simulink model "ZynqBF_2tx_fpga_interface"  (R2018b)
settings: Solver=FixedStepDiscrete  StartTime=0.0  StopTime=inf  RelTol=1e-3  EnableMultiTasking=on
undefined symbols (not defined in the file): Fs, ip
libraries: gm_ZynqBF_2tx_fpga_lib x2, zynqlib x1
settings Model: SimulationMode=external  Creator=jason  LastModifiedBy=meyer
settings SolverCC: ConcurrentTasks=on  PositivePriorityOrder=on
settings DataIOCC: SaveOutput=off  SaveTime=off
settings OptimizationCC: BlockReduction=off  ConditionallyExecuteInputs=off  EnhancedBackFolding=on  PassReuseOutputArgsAs=Individual arguments  MaxStackSize=64  OptimizeBlockOrder=speed  DifferentSizesBufferReuse=on  OptimizationCustomize=off
settings DebuggingCC: AlgebraicLoopMsg=error  SingleTaskRateTransMsg=error  ParameterPrecisionLossMsg=none  ParameterTunabilityLossMsg=error  StrictBusMsg=ErrorOnBusTreatedAsVector
settings HardwareCC: ProdBitPerPointer=32  ProdBitPerSizeT=32  ProdBitPerPtrDiffT=32  ProdLargestAtomicInteger=Long  ProdLargestAtomicFloat=Double  ProdWordSize=32  ProdLongLongMode=on  ProdHWDeviceType=ARM Compatible->ARM Cortex  TargetLargestAtomicInteger=Long  TargetLargestAtomicFloat=Double  TargetIntDivRoundTo=Zero  TargetEndianess=LittleEndian  TargetHWDeviceType=ARM Compatible->ARM Cortex
settings SFSimCC: SimUseLocalCustomCode=off  MATLABDynamicMemAlloc=off
settings RTWCC: SystemTargetFile=ert.tlc  HardwareBoard=Xilinx Zynq-7000 Based IIO Radio  TLCOptions="-aInlineSetEventsForThisBaseRateFcn=TLC_FALSE -aSuppressMultiTaskScheduler=TLC_FALSE  -aRateBasedStepFcn=0"  TemplateMakefile=ert_default_tmf  GenerateReport=on  RTWUseLocalCustomCode=off  Toolchain=Linaro AArch32 Linux v6.3.1  IncludeHyperlinkInReport=on  LaunchReport=on  GenerateTraceInfo=on  GenerateTraceReport=on  GenerateTraceReportSl=on  GenerateTraceReportSf=on  GenerateTraceReportEml=on
settings CodeAppCC: ForceParamTrailComments=on  IgnoreCustomStorageClasses=off  OperatorAnnotations=on  SimulinkDataObjDesc=on  SFDataObjDesc=on  InsertBlockDesc=on

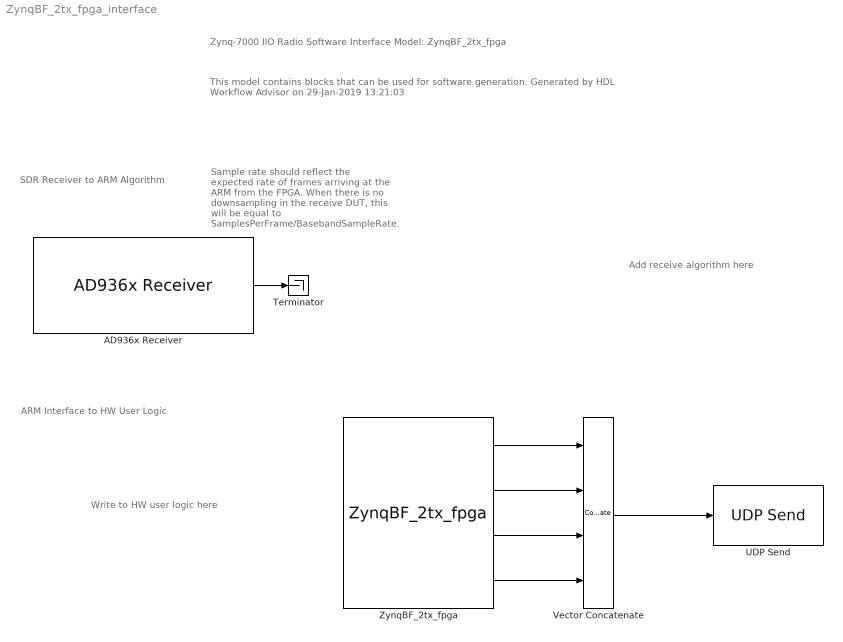
== system ZynqBF_2tx_fpga_interface ==
  note: Zynq-7000 IIO Radio Software Interface Model: ZynqBF_2tx_fpga
  note: This model contains blocks that can be used for software generation.
      |
      | Generated by HDL Workflow Advisor on 29-Jan-2019 13:21:03
  note: SDR Receiver to ARM Algorithm
  note: ARM Interface to HW User Logic
  note: Add receive algorithm here
  note: Write to HW user logic here
  note: Sample rate should reflect the expected rate of frames arriving at the ARM from the FPGA. When there is no downsampling in the receive DUT, this will be equal to SamplesPerFrame/BasebandSampleRate.
  AD936x Receiver : gm_ZynqBF_2tx_fpga_lib/AD936x Receiver  IPAddress=192.168.3.2  uri=ip:10.0.0.200  CenterFrequencySource=Dialog  CenterFrequency=0.9e9  GainSource=AGC Slow Attack  GainSourceBlock=Dialog  Gain=70  ChannelMapping=1  BasebandSampleRate=540.54e3  OutputDataType=double  SamplesPerFrame=200000  OverflowOutputPort=off  EnableBurstMode=on  NumFramesInBurst=1  ShowAdvancedProperties=off  UseCustomFilter=off  filtPathRates=[ 737280000, 11520000, 3840000, 1920000, 960000, 240000 ]  filtCoefficients=round( fir1( 127, 0.75 )*2^15*10^1.2 )  filtCoefficientSize=128  filtDecimInterpFactor=4  filtGain=-12  filtRFBandwidth=18e6  filterConfigStruct=struct()  EnableQuadratureCorrection=on  EnableRFDCCorrection=on  EnableBasebandDCCorrection=on  OverrideSampleTime=off  SampleTime=0.02  DataTimeout=Inf  ENSMPinControlMode=None  BISTLoopbackMode=Disabled  BISTToneInject=Disabled  BISTSignalGen=PRBS  BISTToneFreq=Fs/32  BISTToneLevel=0
  Terminator : Terminator
  UDP Send : zynqlib/UDP Send  remoteURL='192.168.3.1'  remotePort=25000  localURL='255.255.255.255'  localPortSource=Automatically determine  localPort=-1  sampletime=-1  blockPlatform=ZYNQ  separateLengthPort=0
      settings: SourceProductName=Embedded Coder Support Package for Xilinx Zynq Platform  SourceProductBaseCode=ECZYNQ7000
  Vector Concatenate : Concatenate  NumInputs=4
  ZynqBF_2tx_fpga : gm_ZynqBF_2tx_fpga_lib/ZynqBF_2tx_fpga
  wires:
  ZynqBF_2tx_fpga/1 -> Vector Concatenate/1
  ZynqBF_2tx_fpga/2 -> Vector Concatenate/2
  ZynqBF_2tx_fpga/3 -> Vector Concatenate/3
  ZynqBF_2tx_fpga/4 -> Vector Concatenate/4
  Vector Concatenate/1 -> UDP Send/1
  AD936x Receiver/1 -> Terminator/1
